simulink model "aocs_plant"  (R2025a)
settings: Solver=ode45  StartTime=0  StopTime=200  RelTol=1e-09  AbsTol=1e-10
undefined symbols (not defined in the file): AOCS, AOCS_Config, AOCS_EnvironmentConfig, AOCS_GNCConfig, AOCS_OrbitConfig, AOCS_SensorConfig, IAU, juliandate, propagateOnboardSgp4
libraries: aerolibtransform2 x8, simulink x8, matrix_library x5
(part 1 of 3)
settings Model: Creator=aocs-simulation  LastModifiedBy=juliankazmierski
settings DebuggingCC: UnconnectedInputMsg=error  UnconnectedOutputMsg=error  UnconnectedLineMsg=error

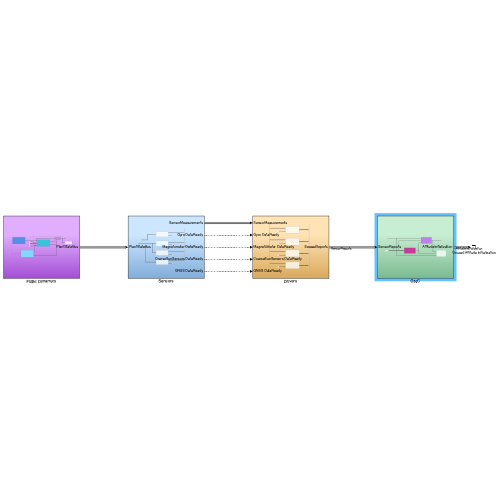
[thumbnail: Simulink's stored preview of the top-level diagram]
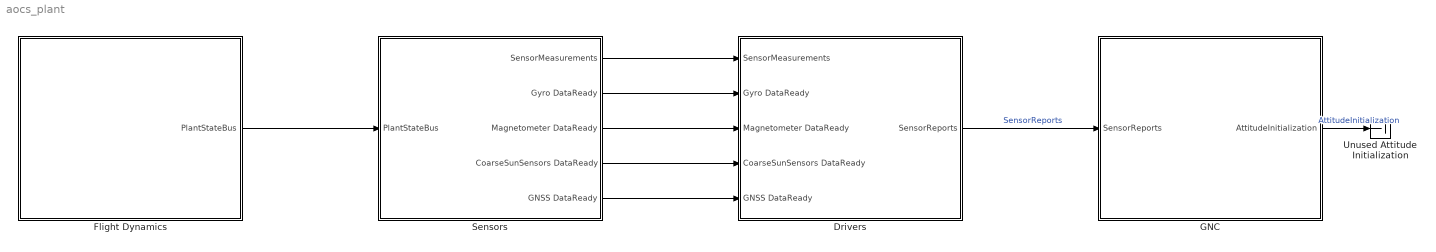
== system aocs_plant ==
  Drivers : Subsystem
  Flight Dynamics : Subsystem
  GNC : Subsystem
  Sensors : Subsystem
  Unused Attitude Initialization : Terminator
  wires:
  Flight Dynamics/1(PlantStateBus) -> Sensors/1(PlantStateBus)
  Sensors/1(SensorMeasurements) -> Drivers/1(SensorMeasurements)
  Sensors/2(Gyro DataReady) -> Drivers/2(Gyro DataReady)
  Sensors/3(Magnetometer DataReady) -> Drivers/3(Magnetometer DataReady)
  Sensors/4(CoarseSunSensors DataReady) -> Drivers/4(CoarseSunSensors DataReady)
  Sensors/5(GNSS DataReady) -> Drivers/5(GNSS DataReady)
  Drivers/1(SensorReports) -> GNC/1(SensorReports)  "SensorReports"
  GNC/1(AttitudeInitialization) -> Unused Attitude Initialization/1  "AttitudeInitialization"

== system aocs_plant/Drivers ==
  SensorMeasurements : Inport  OutDataTypeStr=Bus: SensorMeasurementBus
  Gyro DataReady : Inport  Port=2  OutputFunctionCall=on
  Magnetometer DataReady : Inport  Port=3  OutputFunctionCall=on
  CoarseSunSensors DataReady : Inport  Port=4  OutputFunctionCall=on
  GNSS DataReady : Inport  Port=5  OutputFunctionCall=on
  Coarse Sun Sensors Driver : Subsystem
  GNSS Driver : Subsystem
  Gyro Driver : Subsystem
  Magnetometer Driver : Subsystem
  Select Measurements : BusSelector  OutputSignals=Gyro,Magnetometer,CoarseSunSensors,GNSS
  Sensor Report Bus Assembly : BusCreator  Inputs=4  OutDataTypeStr=Bus: SensorReportBus
  SensorReports : Outport
  wires:
  SensorMeasurements/1 -> Select Measurements/1
  Select Measurements/1 -> Gyro Driver/1(Measurement)  "<Gyro>"
  Gyro DataReady/1 -> Gyro Driver/2(DataReady)
  Select Measurements/2 -> Magnetometer Driver/1(Measurement)  "<Magnetometer>"
  Magnetometer DataReady/1 -> Magnetometer Driver/2(DataReady)
  Select Measurements/3 -> Coarse Sun Sensors Driver/1(Measurement)  "<CoarseSunSensors>"
  CoarseSunSensors DataReady/1 -> Coarse Sun Sensors Driver/2(DataReady)
  Select Measurements/4 -> GNSS Driver/1(Measurement)  "<GNSS>"
  GNSS DataReady/1 -> GNSS Driver/2(DataReady)
  Gyro Driver/1(Report) -> Sensor Report Bus Assembly/1  "Gyro"
  Magnetometer Driver/1(Report) -> Sensor Report Bus Assembly/2  "Magnetometer"
  Coarse Sun Sensors Driver/1(Report) -> Sensor Report Bus Assembly/3  "CoarseSunSensors"
  GNSS Driver/1(Report) -> Sensor Report Bus Assembly/4  "GNSS"
  Sensor Report Bus Assembly/1 -> SensorReports/1

== system aocs_plant/Flight Dynamics ==
  Attitude Dynamics : Subsystem
  Environment Config : Constant  Value=AOCS_EnvironmentConfig  OutDataTypeStr=Bus: EnvironmentConfigBus
  Numerical Checks : Subsystem
  Orbit & Environment : Subsystem
  Orbit Config : Constant  Value=AOCS_OrbitConfig  VectorParams1D=off  OutDataTypeStr=Bus: OrbitConfigBus
  Plant State Bus Creator : BusCreator  Inputs=4  OutDataTypeStr=Bus: PlantStateBus
  Plant Time : Clock
  SpacecraftConfig : Constant  Value=AOCS_Config  OutDataTypeStr=Bus: ConfigBus
  Torque Sum : Subsystem
  PlantStateBus : Outport  OutDataTypeStr=Bus: PlantStateBus
  wires:
  Orbit & Environment/2(EnvironmentBus) -> Torque Sum/2(EnvironmentBus), Plant State Bus Creator/4  "Environment"
  Attitude Dynamics/1(AttitudeState) -> Orbit & Environment/1(AttitudeState), Plant State Bus Creator/3  "AttitudeState"
  Torque Sum/1(Torque_B) -> Attitude Dynamics/1(Torque_B)
  SpacecraftConfig/1 -> Orbit & Environment/4(AocsConfig), Torque Sum/1(Config)
  Environment Config/1 -> Orbit & Environment/3(EnvironmentConfig)
  Orbit Config/1 -> Orbit & Environment/2(OrbitConfig)
  Plant Time/1 -> Plant State Bus Creator/1  "time_s"
  Plant State Bus Creator/1 -> PlantStateBus/1, Numerical Checks/1(PlantState)  "PlantStateBus"
  Orbit & Environment/1(OrbitState) -> Plant State Bus Creator/2  "OrbitState"

== system aocs_plant/GNC ==
  SensorReports : Inport  OutDataTypeStr=Bus: SensorReportBus
  GNC Config : Constant  Value=AOCS_GNCConfig  OutDataTypeStr=Bus: GNCConfigBus
  Onboard Reference Vectors : Subsystem
  Select Initialization Config : BusSelector  OutputSignals=AttitudeInitialization
  State Estimation (MEKF) : Subsystem
  TRIAD Initialization : Subsystem
  AttitudeInitialization : Outport  OutDataTypeStr=Bus: AttitudeInitializationBus
  wires:
  GNC Config/1 -> Select Initialization Config/1
  Select Initialization Config/1 -> Onboard Reference Vectors/1(InitializationConfig), TRIAD Initialization/2(InitializationConfig)  "<AttitudeInitialization>"
  SensorReports/1 -> State Estimation (MEKF)/3(SensorReports), TRIAD Initialization/1(SensorReports)
  Onboard Reference Vectors/1(ReferenceVectors) -> TRIAD Initialization/3(ReferenceVectors), State Estimation (MEKF)/2(ReferenceVectors)  "ReferenceVectors"
  TRIAD Initialization/1(AttitudeInitialization) -> State Estimation (MEKF)/1(AttitudeInitialization), AttitudeInitialization/1  "AttitudeInitialization"

== system aocs_plant/Sensors ==
  PlantStateBus : Inport
  Bus Selector : BusSelector  OutputSignals=AttitudeState,Environment,OrbitState
  Coarse Sun Sensors : Subsystem
  GNSS : Subsystem
  Gyro : Subsystem
  Magnetometer : Subsystem
  Sensor Measurement Bus Assembly : BusCreator  Inputs=4  OutDataTypeStr=Bus: SensorMeasurementBus
  SensorMeasurements : Outport
  Gyro DataReady : Outport  Port=2  OutputFunctionCall=on
  Magnetometer DataReady : Outport  Port=3  OutputFunctionCall=on
  CoarseSunSensors DataReady : Outport  Port=4  OutputFunctionCall=on
  GNSS DataReady : Outport  Port=5  OutputFunctionCall=on
  wires:
  PlantStateBus/1 -> Bus Selector/1
  Bus Selector/1 -> Gyro/1(AttitudeState)  "<AttitudeState>"
  Bus Selector/2 -> Coarse Sun Sensors/1(Environment), Magnetometer/1(Environment)  "<Environment>"
  Gyro/1(Gyro) -> Sensor Measurement Bus Assembly/1  "Gyro"
  Magnetometer/1(Magnetometer) -> Sensor Measurement Bus Assembly/2  "Magnetometer"
  Sensor Measurement Bus Assembly/1 -> SensorMeasurements/1  "SensorMeasurementBus"
  Coarse Sun Sensors/1(CoarseSunSensors) -> Sensor Measurement Bus Assembly/3  "CoarseSunSensors"
  Bus Selector/3 -> GNSS/1(OrbitState)  "<OrbitState>"
  GNSS/1(GNSS) -> Sensor Measurement Bus Assembly/4  "GNSS"
  Gyro/2(DataReady) -> Gyro DataReady/1
  Magnetometer/2(DataReady) -> Magnetometer DataReady/1
  Coarse Sun Sensors/2(DataReady) -> CoarseSunSensors DataReady/1
  GNSS/2(DataReady) -> GNSS DataReady/1

== system aocs_plant/Drivers/Coarse Sun Sensors Driver ==
  Measurement : Inport  OutDataTypeStr=Bus: CoarseSunSensorMeasurementBus
  DataReady : Inport  Port=2  OutputFunctionCall=on
  Receipt Clock : Clock
  Receive Sample : Subsystem
  Report : Outport
  wires:
  Measurement/1 -> Receive Sample/1(Measurement)
  Receipt Clock/1 -> Receive Sample/2(Receipt Time)
  DataReady/1 -> Receive Sample/Trigger
  Receive Sample/1(Report) -> Report/1

== system aocs_plant/Drivers/GNSS Driver ==
  Measurement : Inport  OutDataTypeStr=Bus: GnssMeasurementBus
  DataReady : Inport  Port=2  OutputFunctionCall=on
  Receipt Clock : Clock
  Receive Sample : Subsystem
  Report : Outport
  wires:
  Measurement/1 -> Receive Sample/1(Measurement)
  Receipt Clock/1 -> Receive Sample/2(Receipt Time)
  DataReady/1 -> Receive Sample/Trigger
  Receive Sample/1(Report) -> Report/1

== system aocs_plant/Drivers/Gyro Driver ==
  Measurement : Inport  OutDataTypeStr=Bus: GyroMeasurementBus
  DataReady : Inport  Port=2  OutputFunctionCall=on
  Receipt Clock : Clock
  Receive Sample : Subsystem
  Report : Outport
  wires:
  Measurement/1 -> Receive Sample/1(Measurement)
  Receipt Clock/1 -> Receive Sample/2(Receipt Time)
  DataReady/1 -> Receive Sample/Trigger
  Receive Sample/1(Report) -> Report/1

== system aocs_plant/Drivers/Magnetometer Driver ==
  Measurement : Inport  OutDataTypeStr=Bus: MagnetometerMeasurementBus
  DataReady : Inport  Port=2  OutputFunctionCall=on
  Receipt Clock : Clock
  Receive Sample : Subsystem
  Report : Outport
  wires:
  Measurement/1 -> Receive Sample/1(Measurement)
  Receipt Clock/1 -> Receive Sample/2(Receipt Time)
  DataReady/1 -> Receive Sample/Trigger
  Receive Sample/1(Report) -> Report/1

== system aocs_plant/Flight Dynamics/Attitude Dynamics ==
  Torque_B : Inport
  6DOF (Quaternion) : EOM6DOFBodyQuat  eul_0=AOCS_Config.euler_BI_0_rad  pm_0=AOCS_Config.omega_BI_B_0  mass_0=3.71  inertia=AOCS_Config.I_B
  Bus Creator : BusCreator  Inputs=4
  Terminator : Terminator
  Terminator1 : Terminator
  Terminator2 : Terminator
  Zero_Forces : Constant  Value=[0;0;0]
  AttitudeState : Outport  OutDataTypeStr=Bus: AttitudeStateBus
  wires:
  Torque_B/1 -> 6DOF (Quaternion)/2
  Zero_Forces/1 -> 6DOF (Quaternion)/1
  6DOF (Quaternion)/1 -> Terminator/1
  6DOF (Quaternion)/2 -> Terminator1/1
  6DOF (Quaternion)/6 -> Terminator2/1
  6DOF (Quaternion)/3 -> Bus Creator/1  "euler_rad"
  6DOF (Quaternion)/5 -> Bus Creator/3  "DCM_be"
  6DOF (Quaternion)/7 -> Bus Creator/4  "omega_b"
  Bus Creator/1 -> AttitudeState/1
  6DOF (Quaternion)/4 -> Bus Creator/2  "q_be"

== system aocs_plant/Flight Dynamics/Numerical Checks ==
  PlantState : Inport  OutDataTypeStr=Bus: PlantStateBus
  Finite Plant State : Assertion
  Finite Values : MATLAB Function  TreatAsAtomicUnit=on
  wires:
  PlantState/1 -> Finite Values/1(state)
  Finite Values/1(ok) -> Finite Plant State/1

== system aocs_plant/Flight Dynamics/Orbit & Environment ==
  AttitudeState : Inport
  OrbitConfig : Inport  Port=2
  EnvironmentConfig : Inport  Port=3
  AocsConfig : Inport  Port=4
  Disturbance Torques : Subsystem
  Environment Bus Assembly : Subsystem
  Environment Products : Subsystem
  Orbit Propagator & Time : Subsystem
  OrbitState : Outport  OutDataTypeStr=Bus: OrbitStateBus
  EnvironmentBus : Outport  Port=2  OutDataTypeStr=Bus: EnvironmentBus
  wires:
  AocsConfig/1 -> Disturbance Torques/1(AocsConfig)  "AocsConfig"
  Disturbance Torques/1(Disturbance) -> Environment Bus Assembly/1(Disturbance)  "Disturbance"
  Environment Bus Assembly/1(EnvironmentBus) -> EnvironmentBus/1  "EnvironmentBus"
  Environment Products/2(MagneticField) -> Environment Bus Assembly/2(MagneticField), Disturbance Torques/7(MagneticField)
  AttitudeState/1 -> Disturbance Torques/3(AttitudeState), Environment Products/2(AttitudeState)  "AttitudeState"
  Orbit Propagator & Time/1(OrbitState) -> OrbitState/1, Disturbance Torques/4(OrbitState), Environment Products/3(OrbitState)
  Orbit Propagator & Time/2(EnvironmentContext) -> Disturbance Torques/5(EnvironmentContext), Environment Products/4(EnvironmentContext)
  EnvironmentConfig/1 -> Environment Products/1(EnvironmentConfig), Disturbance Torques/2(EnvironmentConfig)  "EnvironmentConfig"
  Environment Products/1(SRP) -> Disturbance Torques/6(SRP)
  Environment Products/4(Illumination) -> Environment Bus Assembly/4(Illumination)
  Environment Products/3(Sun) -> Environment Bus Assembly/3(Sun)
  OrbitConfig/1 -> Orbit Propagator & Time/1(OrbitConfig)  "OrbitConfig"
  Environment Products/5(Atmosphere) -> Disturbance Torques/8(Atmosphere), Environment Bus Assembly/5(Atmosphere)
  Disturbance Torques/2(OrbitAcceleration) -> Orbit Propagator & Time/2(OrbitAcceleration)

== system aocs_plant/Flight Dynamics/Torque Sum ==
  Config : Inport
  EnvironmentBus : Inport  Port=2
  Add : Sum
  Bus Selector : BusSelector  OutputSignals=M_dist_B_Nm
  Bus Selector1 : BusSelector  OutputSignals=M_ext_B
  Torque_B : Outport
  wires:
  EnvironmentBus/1 -> Bus Selector/1
  Bus Selector/1 -> Add/1  "<M_dist_B_Nm>"
  Add/1 -> Torque_B/1
  Config/1 -> Bus Selector1/1
  Bus Selector1/1 -> Add/2  "<M_ext_B>"

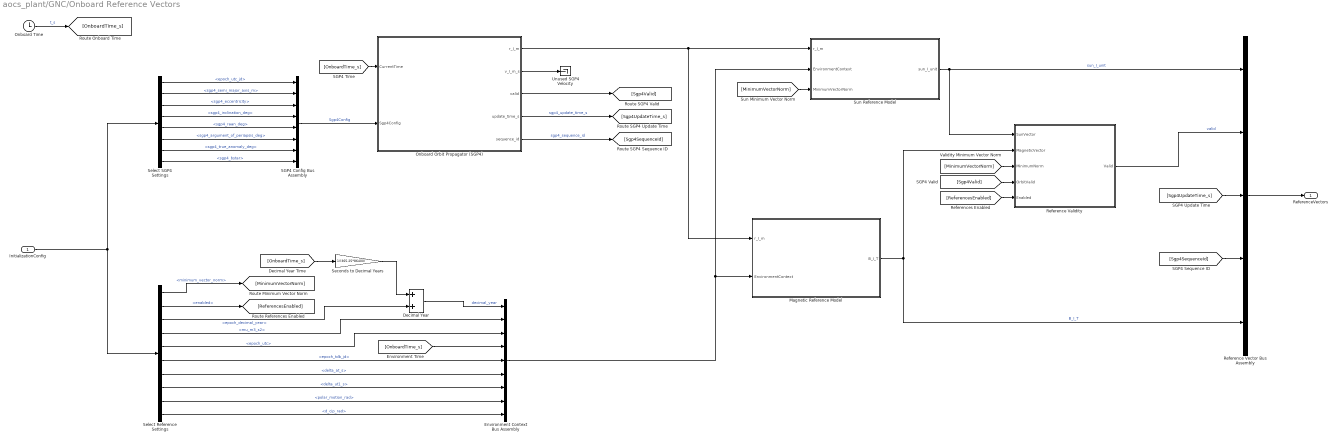
== system aocs_plant/GNC/Onboard Reference Vectors ==
  InitializationConfig : Inport  OutDataTypeStr=Bus: AttitudeInitializationConfigBus
  Decimal Year : Sum
  Environment Context Bus Assembly : BusCreator  Inputs=9  OutDataTypeStr=Bus: EnvironmentContextBus
  Magnetic Reference Model : Subsystem
  Onboard Orbit Propagator (SGP4) : Subsystem
  Onboard Time : Clock
  Reference Validity : Subsystem
  Reference Vector Bus Assembly : BusCreator  Inputs=5  OutDataTypeStr=Bus: ReferenceVectorBus
  SGP4 Config Bus Assembly : BusCreator  Inputs=8  OutDataTypeStr=Bus: Sgp4ConfigBus  NonVirtualBus=on
  Seconds to Decimal Years : Gain  Gain=1/(365.25*86400)
  Select Reference Settings : BusSelector  OutputSignals=minimum_vector_norm,enabled,epoch_decimal_year,mu_m3_s2,epoch_utc,epoch_tdb_jd,delta_at_s,delta_ut1_s,polar_motion_rad,d_cip_rad
  Select SGP4 Settings : BusSelector  OutputSignals=epoch_utc_jd,sgp4_semi_major_axis_m,sgp4_eccentricity,sgp4_inclination_deg,sgp4_raan_deg,sgp4_argument_of_periapsis_deg,sgp4_true_anomaly_deg,sgp4_bstar
  Sun Reference Model : Subsystem
  Unused SGP4 Velocity : Terminator
  ReferenceVectors : Outport  OutDataTypeStr=Bus: ReferenceVectorBus
  wires:
  InitializationConfig/1 -> Select Reference Settings/1, Select SGP4 Settings/1
  Onboard Time/1 -> [OnboardTime_s]  "t_s"
  Select SGP4 Settings/1 -> SGP4 Config Bus Assembly/1  "<epoch_utc_jd>"
  Select SGP4 Settings/2 -> SGP4 Config Bus Assembly/2  "<sgp4_semi_major_axis_m>"
  Select SGP4 Settings/3 -> SGP4 Config Bus Assembly/3  "<sgp4_eccentricity>"
  Select SGP4 Settings/4 -> SGP4 Config Bus Assembly/4  "<sgp4_inclination_deg>"
  Select SGP4 Settings/5 -> SGP4 Config Bus Assembly/5  "<sgp4_raan_deg>"
  Select SGP4 Settings/6 -> SGP4 Config Bus Assembly/6  "<sgp4_argument_of_periapsis_deg>"
  Select SGP4 Settings/7 -> SGP4 Config Bus Assembly/7  "<sgp4_true_anomaly_deg>"
  Select SGP4 Settings/8 -> SGP4 Config Bus Assembly/8  "<sgp4_bstar>"
  [OnboardTime_s] -> Onboard Orbit Propagator (SGP4)/1(CurrentTime)
  SGP4 Config Bus Assembly/1 -> Onboard Orbit Propagator (SGP4)/2(Sgp4Config)  "Sgp4Config"
  Select Reference Settings/1 -> [MinimumVectorNorm]  "<minimum_vector_norm>"
  Select Reference Settings/2 -> [ReferencesEnabled]  "<enabled>"
  Select Reference Settings/3 -> Decimal Year/2  "<epoch_decimal_year>"
  Select Reference Settings/4 -> Environment Context Bus Assembly/2  "<mu_m3_s2>"
  Select Reference Settings/5 -> Environment Context Bus Assembly/3  "<epoch_utc>"
  Select Reference Settings/6 -> Environment Context Bus Assembly/5  "<epoch_tdb_jd>"
  Select Reference Settings/7 -> Environment Context Bus Assembly/6  "<delta_at_s>"
  Select Reference Settings/8 -> Environment Context Bus Assembly/7  "<delta_ut1_s>"
  Select Reference Settings/9 -> Environment Context Bus Assembly/8  "<polar_motion_rad>"
  Select Reference Settings/10 -> Environment Context Bus Assembly/9  "<d_cip_rad>"
  [OnboardTime_s] -> Seconds to Decimal Years/1
  Seconds to Decimal Years/1 -> Decimal Year/1
  Decimal Year/1 -> Environment Context Bus Assembly/1  "decimal_year"
  [OnboardTime_s] -> Environment Context Bus Assembly/4
  Onboard Orbit Propagator (SGP4)/1(r_I_m) -> Sun Reference Model/1(r_I_m), Magnetic Reference Model/1(r_I_m)
  Onboard Orbit Propagator (SGP4)/2(v_I_m_s) -> Unused SGP4 Velocity/1
  Onboard Orbit Propagator (SGP4)/3(valid) -> [Sgp4Valid]
  Onboard Orbit Propagator (SGP4)/4(update_time_s) -> [Sgp4UpdateTime_s]  "sgp4_update_time_s"
  Onboard Orbit Propagator (SGP4)/5(sequence_id) -> [Sgp4SequenceId]  "sgp4_sequence_id"
  Environment Context Bus Assembly/1 -> Magnetic Reference Model/2(EnvironmentContext), Sun Reference Model/2(EnvironmentContext)
  [MinimumVectorNorm] -> Sun Reference Model/3(MinimumVectorNorm)
  Sun Reference Model/1(sun_I_unit) -> Reference Validity/1(SunVector), Reference Vector Bus Assembly/1  "sun_I_unit"
  Magnetic Reference Model/1(B_I_T) -> Reference Vector Bus Assembly/5, Reference Validity/2(MagneticVector)  "B_I_T"
  [MinimumVectorNorm] -> Reference Validity/3(MinimumNorm)
  [Sgp4Valid] -> Reference Validity/4(OrbitValid)
  [ReferencesEnabled] -> Reference Validity/5(Enabled)
  Reference Validity/1(Valid) -> Reference Vector Bus Assembly/2  "valid"
  [Sgp4UpdateTime_s] -> Reference Vector Bus Assembly/3
  [Sgp4SequenceId] -> Reference Vector Bus Assembly/4
  Reference Vector Bus Assembly/1 -> ReferenceVectors/1

== system aocs_plant/GNC/State Estimation (MEKF) ==
  note: Reserved for the six-state multiplicative EKF: attitude error plus gyro bias.
  AttitudeInitialization : Inport  OutDataTypeStr=Bus: AttitudeInitializationBus
  ReferenceVectors : Inport  Port=2  OutDataTypeStr=Bus: ReferenceVectorBus
  SensorReports : Inport  Port=3  OutDataTypeStr=Bus: SensorReportBus
  Unused AttitudeInitialization : Terminator
  Unused ReferenceVectors : Terminator
  Unused SensorReports : Terminator
  wires:
  SensorReports/1 -> Unused SensorReports/1
  ReferenceVectors/1 -> Unused ReferenceVectors/1
  AttitudeInitialization/1 -> Unused AttitudeInitialization/1

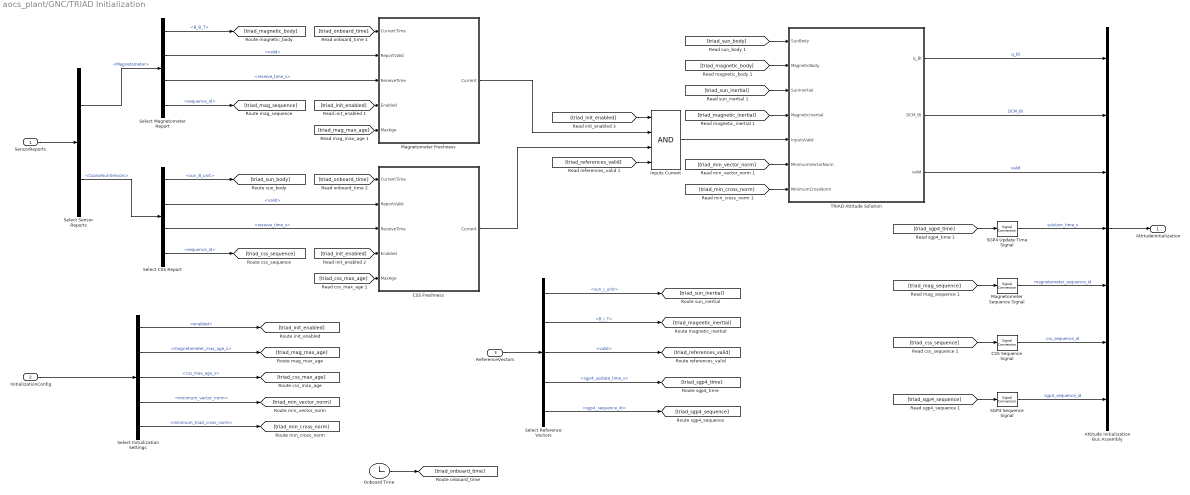
== system aocs_plant/GNC/TRIAD Initialization ==
  SensorReports : Inport  OutDataTypeStr=Bus: SensorReportBus
  InitializationConfig : Inport  Port=2  OutDataTypeStr=Bus: AttitudeInitializationConfigBus
  ReferenceVectors : Inport  Port=3  OutDataTypeStr=Bus: ReferenceVectorBus
  Attitude Initialization Bus Assembly : BusCreator  Inputs=7  OutDataTypeStr=Bus: AttitudeInitializationBus
  CSS Freshness : Subsystem
  CSS Sequence Signal : SignalConversion  OverrideOpt=off
  Inputs Current : Logic  Inputs=4  AllPortsSameDT=off  OutDataTypeStr=boolean
  Magnetometer Freshness : Subsystem
  Magnetometer Sequence Signal : SignalConversion  OverrideOpt=off
  Onboard Time : Clock
  SGP4 Sequence Signal : SignalConversion  OverrideOpt=off
  SGP4 Update Time Signal : SignalConversion  OverrideOpt=off
  Select CSS Report : BusSelector  OutputSignals=sun_B_unit,valid,receive_time_s,sequence_id
  Select Initialization Settings : BusSelector  OutputSignals=enabled,magnetometer_max_age_s,css_max_age_s,minimum_vector_norm,minimum_triad_cross_norm
  Select Magnetometer Report : BusSelector  OutputSignals=B_B_T,valid,receive_time_s,sequence_id
  Select Reference Vectors : BusSelector  OutputSignals=sun_I_unit,B_I_T,valid,sgp4_update_time_s,sgp4_sequence_id
  Select Sensor Reports : BusSelector  OutputSignals=Magnetometer,CoarseSunSensors
  TRIAD Attitude Solution : Subsystem
  AttitudeInitialization : Outport  OutDataTypeStr=Bus: AttitudeInitializationBus
  wires:
  SensorReports/1 -> Select Sensor Reports/1
  Select Sensor Reports/1 -> Select Magnetometer Report/1  "<Magnetometer>"
  Select Sensor Reports/2 -> Select CSS Report/1  "<CoarseSunSensors>"
  ReferenceVectors/1 -> Select Reference Vectors/1
  InitializationConfig/1 -> Select Initialization Settings/1
  Select Magnetometer Report/2 -> Magnetometer Freshness/2(ReportValid)  "<valid>"
  Select Magnetometer Report/3 -> Magnetometer Freshness/3(ReceiveTime)  "<receive_time_s>"
  Select CSS Report/2 -> CSS Freshness/2(ReportValid)  "<valid>"
  Select CSS Report/3 -> CSS Freshness/3(ReceiveTime)  "<receive_time_s>"
  Magnetometer Freshness/1(Current) -> Inputs Current/2
  CSS Freshness/1(Current) -> Inputs Current/3
  Inputs Current/1 -> TRIAD Attitude Solution/5(InputsValid)
  TRIAD Attitude Solution/1(q_BI) -> Attitude Initialization Bus Assembly/1  "q_BI"
  TRIAD Attitude Solution/2(DCM_BI) -> Attitude Initialization Bus Assembly/2  "DCM_BI"
  TRIAD Attitude Solution/3(valid) -> Attitude Initialization Bus Assembly/3  "valid"
  SGP4 Update Time Signal/1 -> Attitude Initialization Bus Assembly/4  "solution_time_s"
  Magnetometer Sequence Signal/1 -> Attitude Initialization Bus Assembly/5  "magnetometer_sequence_id"
  CSS Sequence Signal/1 -> Attitude Initialization Bus Assembly/6  "css_sequence_id"
  SGP4 Sequence Signal/1 -> Attitude Initialization Bus Assembly/7  "sgp4_sequence_id"
  Attitude Initialization Bus Assembly/1 -> AttitudeInitialization/1
  Select Magnetometer Report/1 -> [triad_magnetic_body]  "<B_B_T>"
  [triad_magnetic_body] -> TRIAD Attitude Solution/2(MagneticBody)
  Select Magnetometer Report/4 -> [triad_mag_sequence]  "<sequence_id>"
  [triad_mag_sequence] -> Magnetometer Sequence Signal/1
  Select CSS Report/1 -> [triad_sun_body]  "<sun_B_unit>"
  [triad_sun_body] -> TRIAD Attitude Solution/1(SunBody)
  Select CSS Report/4 -> [triad_css_sequence]  "<sequence_id>"
  [triad_css_sequence] -> CSS Sequence Signal/1
  Select Initialization Settings/1 -> [triad_init_enabled]  "<enabled>"
  [triad_init_enabled] -> Magnetometer Freshness/4(Enabled)
  [triad_init_enabled] -> CSS Freshness/4(Enabled)
  [triad_init_enabled] -> Inputs Current/1
  Select Initialization Settings/2 -> [triad_mag_max_age]  "<magnetometer_max_age_s>"
  [triad_mag_max_age] -> Magnetometer Freshness/5(MaxAge)
  Select Initialization Settings/3 -> [triad_css_max_age]  "<css_max_age_s>"
  [triad_css_max_age] -> CSS Freshness/5(MaxAge)
  Select Initialization Settings/4 -> [triad_min_vector_norm]  "<minimum_vector_norm>"
  [triad_min_vector_norm] -> TRIAD Attitude Solution/6(MinimumVectorNorm)
  Select Initialization Settings/5 -> [triad_min_cross_norm]  "<minimum_triad_cross_norm>"
  [triad_min_cross_norm] -> TRIAD Attitude Solution/7(MinimumCrossNorm)
  Select Reference Vectors/1 -> [triad_sun_inertial]  "<sun_I_unit>"
  [triad_sun_inertial] -> TRIAD Attitude Solution/3(SunInertial)
  Select Reference Vectors/2 -> [triad_magnetic_inertial]  "<B_I_T>"
  [triad_magnetic_inertial] -> TRIAD Attitude Solution/4(MagneticInertial)
  Select Reference Vectors/3 -> [triad_references_valid]  "<valid>"
  [triad_references_valid] -> Inputs Current/4
  Select Reference Vectors/4 -> [triad_sgp4_time]  "<sgp4_update_time_s>"
  [triad_sgp4_time] -> SGP4 Update Time Signal/1
  Select Reference Vectors/5 -> [triad_sgp4_sequence]  "<sgp4_sequence_id>"
  [triad_sgp4_sequence] -> SGP4 Sequence Signal/1
  Onboard Time/1 -> [triad_onboard_time]
  [triad_onboard_time] -> Magnetometer Freshness/1(CurrentTime)
  [triad_onboard_time] -> CSS Freshness/1(CurrentTime)

== system aocs_plant/Sensors/Coarse Sun Sensors ==
  Environment : Inport
  Bus Selector : BusSelector  OutputSignals=sun_B_unit,solar_flux_shadowed_W_m2,sun_visibility
  CSS Measurement Bus Assembly : BusCreator  Inputs=4  OutDataTypeStr=Bus: CoarseSunSensorMeasurementBus
  Coarse Sun Sensor Model : MATLAB Function  TreatAsAtomicUnit=on
  CssConfig : Constant  Value=AOCS_SensorConfig.CoarseSunSensors  OutDataTypeStr=Bus: CoarseSunSensorConfigBus
  DataReady Generator : FunctionCallGenerator  SampleTime=AOCS_SensorConfig.CoarseSunSensors.sample_time_s
  Measurement Sample Hold : ZeroOrderHold  SampleTime=AOCS_SensorConfig.CoarseSunSensors.sample_time_s
  W : RandomNumber  Mean=zeros(6,1)  Variance=ones(6,1)  Seed=AOCS_SensorConfig.CoarseSunSensors.noise_seed  SampleTime=AOCS_SensorConfig.CoarseSunSensors.sample_time_s
  CoarseSunSensors : Outport
  DataReady : Outport  Port=2  OutputFunctionCall=on
  wires:
  Environment/1 -> Bus Selector/1
  Bus Selector/1 -> Coarse Sun Sensor Model/1(sun_B_unit)  "<sun_B_unit>"
  Bus Selector/2 -> Coarse Sun Sensor Model/2(solar_flux_shadowed_W_m2)  "<solar_flux_shadowed_W_m2>"
  Bus Selector/3 -> Coarse Sun Sensor Model/3(sun_visibility)  "<sun_visibility>"
  CssConfig/1 -> Coarse Sun Sensor Model/4(css)  "css"
  W/1 -> Coarse Sun Sensor Model/5(noise_unit)  "noise_unit"
  Coarse Sun Sensor Model/1(sun_B_unit_meas) -> CSS Measurement Bus Assembly/1  "sun_B_unit"
  Coarse Sun Sensor Model/2(irradiance_W_m2) -> CSS Measurement Bus Assembly/2  "irradiance_W_m2"
  Coarse Sun Sensor Model/3(panel_signals_W_m2) -> CSS Measurement Bus Assembly/3  "panel_signals_W_m2"
  Coarse Sun Sensor Model/4(valid) -> CSS Measurement Bus Assembly/4  "valid"
  CSS Measurement Bus Assembly/1 -> Measurement Sample Hold/1  "CoarseSunSensors"
  Measurement Sample Hold/1 -> CoarseSunSensors/1
  DataReady Generator/1 -> DataReady/1

== system aocs_plant/Sensors/GNSS ==
  OrbitState : Inport
  DataReady Generator : FunctionCallGenerator  SampleTime=AOCS_SensorConfig.GNSS.sample_time_s
  Fix Availability : Subsystem
  GNSS Measurement Bus Assembly : BusCreator  Inputs=3  OutDataTypeStr=Bus: GnssMeasurementBus
  GnssConfig : Constant  Value=AOCS_SensorConfig.GNSS  OutDataTypeStr=Bus: GnssConfigBus
  Measurement Sample Hold : ZeroOrderHold  SampleTime=AOCS_SensorConfig.GNSS.sample_time_s
  Output Selection : Subsystem
  PVT Error Model : Subsystem
  Position Quantizer : Quantizer  QuantizationInterval=AOCS_SensorConfig.GNSS.position_resolution_m
  Position Sample Hold : ZeroOrderHold  SampleTime=AOCS_SensorConfig.GNSS.sample_time_s
  Select Orbit State : BusSelector  OutputSignals=r_I_m,v_I_m_s
  Velocity Quantizer : Quantizer  QuantizationInterval=AOCS_SensorConfig.GNSS.velocity_resolution_m_s
  Velocity Sample Hold : ZeroOrderHold  SampleTime=AOCS_SensorConfig.GNSS.sample_time_s
  GNSS : Outport
  DataReady : Outport  Port=2  OutputFunctionCall=on
  wires:
  OrbitState/1 -> Select Orbit State/1  "OrbitState"
  Select Orbit State/1 -> Position Sample Hold/1  "<r_I_m>"
  Select Orbit State/2 -> Velocity Sample Hold/1  "<v_I_m_s>"
  Position Sample Hold/1 -> PVT Error Model/1(rTruth_I_m)
  Velocity Sample Hold/1 -> PVT Error Model/2(vTruth_I_m_s)
  PVT Error Model/1(rMeasured_I_m) -> Position Quantizer/1
  PVT Error Model/2(vMeasured_I_m_s) -> Velocity Quantizer/1
  Position Quantizer/1 -> Output Selection/1(rNominal_I_m)  "r_I_m_nominal"
  Velocity Quantizer/1 -> Output Selection/2(vNominal_I_m_s)  "v_I_m_s_nominal"
  GnssConfig/1 -> Fix Availability/1(GnssConfig), Output Selection/3(GnssConfig)  "GNSSConfig"
  Fix Availability/1(fix_available) -> Output Selection/4(fix_available)  "fix_available"
  Output Selection/1(r_I_m) -> GNSS Measurement Bus Assembly/1  "r_I_m"
  Output Selection/2(v_I_m_s) -> GNSS Measurement Bus Assembly/2  "v_I_m_s"
  Output Selection/3(valid) -> GNSS Measurement Bus Assembly/3  "valid"
  GNSS Measurement Bus Assembly/1 -> Measurement Sample Hold/1  "GNSS"
  Measurement Sample Hold/1 -> GNSS/1
  DataReady Generator/1 -> DataReady/1

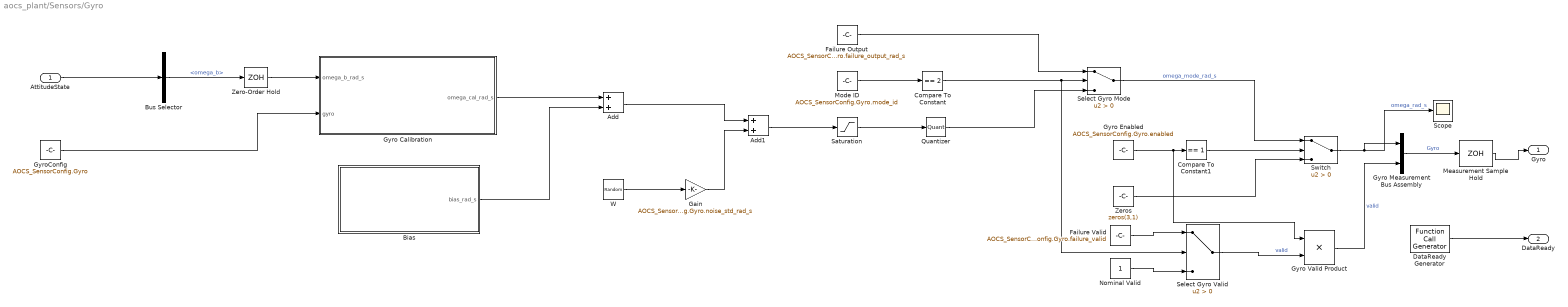
== system aocs_plant/Sensors/Gyro ==
  AttitudeState : Inport
  Add : Sum
  Add1 : Sum
  Bias : Subsystem
  Bus Selector : BusSelector  OutputSignals=omega_b
  Compare To Constant : simulink/Logic and Bit Operations/Compare To Constant  relop===  const=2  OutDataTypeStr=boolean
  Compare To Constant1 : simulink/Logic and Bit Operations/Compare To Constant  relop===  const=1  OutDataTypeStr=boolean
  DataReady Generator : FunctionCallGenerator  SampleTime=AOCS_SensorConfig.Gyro.gyro_sample_time_s
  Failure Output : Constant  Value=AOCS_SensorConfig.Gyro.failure_output_rad_s
  Failure Valid : Constant  Value=AOCS_SensorConfig.Gyro.failure_valid
  Gain : Gain  Gain=AOCS_SensorConfig.Gyro.noise_std_rad_s
  Gyro Calibration : MATLAB Function  TreatAsAtomicUnit=on
  Gyro Enabled : Constant  Value=AOCS_SensorConfig.Gyro.enabled
  Gyro Measurement Bus Assembly : BusCreator  Inputs=2  OutDataTypeStr=Bus: GyroMeasurementBus
  Gyro Valid Product : Product  Inputs=**
  GyroConfig : Constant  Value=AOCS_SensorConfig.Gyro  OutDataTypeStr=Bus: GyroConfigBus
  Measurement Sample Hold : ZeroOrderHold  SampleTime=AOCS_SensorConfig.Gyro.gyro_sample_time_s
  Mode ID : Constant  Value=AOCS_SensorConfig.Gyro.mode_id
  Nominal Valid : Constant
  Quantizer : Quantizer  QuantizationInterval=AOCS_SensorConfig.Gyro.resolution_rad_s
  Saturation : Saturate  UpperLimit=AOCS_SensorConfig.Gyro.range_rad_s  LowerLimit=-AOCS_SensorConfig.Gyro.range_rad_s
  Scope : Scope
      settings: ActiveDisplayYMinimum=1.4855983316703409  ActiveDisplayYMaximum=1.511725104472023
  Select Gyro Mode : Switch  Criteria=u2 > Threshold  SaturateOnIntegerOverflow=off  InputSameDT=off
  Select Gyro Valid : Switch  Criteria=u2 > Threshold  SaturateOnIntegerOverflow=off  InputSameDT=off
  Switch : Switch  Criteria=u2 > Threshold  SaturateOnIntegerOverflow=off  InputSameDT=off
  W : RandomNumber  Seed=AOCS_SensorConfig.Gyro.noise_seed  SampleTime=AOCS_SensorConfig.Gyro.gyro_sample_time_s
  Zero-Order Hold : ZeroOrderHold  SampleTime=AOCS_SensorConfig.Gyro.gyro_sample_time_s
  Zeros : Constant  Value=zeros(3,1)
  Gyro : Outport
  DataReady : Outport  Port=2  OutputFunctionCall=on
  wires:
  AttitudeState/1 -> Bus Selector/1
  Bus Selector/1 -> Zero-Order Hold/1  "<omega_b>"
  Zero-Order Hold/1 -> Gyro Calibration/1(omega_b_rad_s)
  GyroConfig/1 -> Gyro Calibration/2(gyro)
  Gyro Calibration/1(omega_cal_rad_s) -> Add/1
  Bias/1(bias_rad_s) -> Add/2
  W/1 -> Gain/1
  Gain/1 -> Add1/2
  Add/1 -> Add1/1
  Add1/1 -> Saturation/1
  Saturation/1 -> Quantizer/1
  Mode ID/1 -> Compare To Constant/1
  Compare To Constant/1 -> Select Gyro Mode/2, Select Gyro Valid/2
  Failure Output/1 -> Select Gyro Mode/1
  Quantizer/1 -> Select Gyro Mode/3
  Select Gyro Mode/1 -> Switch/1  "omega_mode_rad_s"
  Gyro Enabled/1 -> Compare To Constant1/1, Gyro Valid Product/1
  Compare To Constant1/1 -> Switch/2
  Zeros/1 -> Switch/3
  Switch/1 -> Scope/1, Gyro Measurement Bus Assembly/1  "omega_rad_s"
  Failure Valid/1 -> Select Gyro Valid/1
  Nominal Valid/1 -> Select Gyro Valid/3
  Select Gyro Valid/1 -> Gyro Valid Product/2  "valid"
  Gyro Valid Product/1 -> Gyro Measurement Bus Assembly/2  "valid"
  Gyro Measurement Bus Assembly/1 -> Measurement Sample Hold/1  "Gyro"
  Measurement Sample Hold/1 -> Gyro/1
  DataReady Generator/1 -> DataReady/1

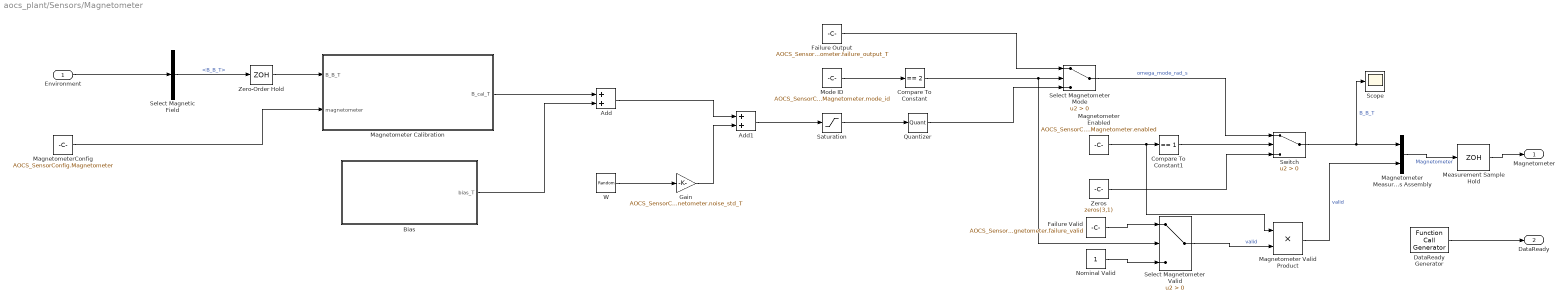
== system aocs_plant/Sensors/Magnetometer ==
  Environment : Inport
  Add : Sum
  Add1 : Sum
  Bias : Subsystem
  Compare To Constant : simulink/Logic and Bit Operations/Compare To Constant  relop===  const=2  OutDataTypeStr=boolean
  Compare To Constant1 : simulink/Logic and Bit Operations/Compare To Constant  relop===  const=1  OutDataTypeStr=boolean
  DataReady Generator : FunctionCallGenerator  SampleTime=AOCS_SensorConfig.Magnetometer.sample_time_s
  Failure Output : Constant  Value=AOCS_SensorConfig.Magnetometer.failure_output_T
  Failure Valid : Constant  Value=AOCS_SensorConfig.Magnetometer.failure_valid
  Gain : Gain  Gain=AOCS_SensorConfig.Magnetometer.noise_std_T
  Magnetometer Calibration : MATLAB Function  TreatAsAtomicUnit=on
  Magnetometer Enabled : Constant  Value=AOCS_SensorConfig.Magnetometer.enabled
  Magnetometer Measurement Bus Assembly : BusCreator  Inputs=2  OutDataTypeStr=Bus: MagnetometerMeasurementBus
  Magnetometer Valid Product : Product  Inputs=**
  MagnetometerConfig : Constant  Value=AOCS_SensorConfig.Magnetometer  OutDataTypeStr=Bus: MagnetometerConfigBus
  Measurement Sample Hold : ZeroOrderHold  SampleTime=AOCS_SensorConfig.Magnetometer.sample_time_s
  Mode ID : Constant  Value=AOCS_SensorConfig.Magnetometer.mode_id
  Nominal Valid : Constant
  Quantizer : Quantizer  QuantizationInterval=AOCS_SensorConfig.Magnetometer.resolution_T
  Saturation : Saturate  UpperLimit=AOCS_SensorConfig.Magnetometer.range_T  LowerLimit=-AOCS_SensorConfig.Magnetometer.range_T
  Scope : Scope
      settings: ActiveDisplayYMinimum=0.99973136391270112  ActiveDisplayYMaximum=1.0056523225715319
  Select Magnetic Field : BusSelector  OutputSignals=B_B_T
  Select Magnetometer Mode : Switch  Criteria=u2 > Threshold  SaturateOnIntegerOverflow=off  InputSameDT=off
  Select Magnetometer Valid : Switch  Criteria=u2 > Threshold  SaturateOnIntegerOverflow=off  InputSameDT=off
  Switch : Switch  Criteria=u2 > Threshold  SaturateOnIntegerOverflow=off  InputSameDT=off
  W : RandomNumber  Seed=AOCS_SensorConfig.Magnetometer.noise_seed  SampleTime=AOCS_SensorConfig.Magnetometer.sample_time_s
  Zero-Order Hold : ZeroOrderHold  SampleTime=AOCS_SensorConfig.Magnetometer.sample_time_s
  Zeros : Constant  Value=zeros(3,1)
  Magnetometer : Outport
  DataReady : Outport  Port=2  OutputFunctionCall=on
  wires:
  Magnetometer Valid Product/1 -> Magnetometer Measurement Bus Assembly/2  "valid"
  Select Magnetometer Valid/1 -> Magnetometer Valid Product/2  "valid"
  Nominal Valid/1 -> Select Magnetometer Valid/3
  Failure Valid/1 -> Select Magnetometer Valid/1
  Zeros/1 -> Switch/3
  Compare To Constant1/1 -> Switch/2
  Magnetometer Enabled/1 -> Magnetometer Valid Product/1, Compare To Constant1/1
  Select Magnetometer Mode/1 -> Switch/1  "omega_mode_rad_s"
  Quantizer/1 -> Select Magnetometer Mode/3
  Failure Output/1 -> Select Magnetometer Mode/1
  Compare To Constant/1 -> Select Magnetometer Valid/2, Select Magnetometer Mode/2
  Mode ID/1 -> Compare To Constant/1
  Saturation/1 -> Quantizer/1
  Add1/1 -> Saturation/1
  Add/1 -> Add1/1
  Gain/1 -> Add1/2
  W/1 -> Gain/1
  Bias/1(bias_T) -> Add/2
  Magnetometer Calibration/1(B_cal_T) -> Add/1
  MagnetometerConfig/1 -> Magnetometer Calibration/2(magnetometer)
  Zero-Order Hold/1 -> Magnetometer Calibration/1(B_B_T)
  Select Magnetic Field/1 -> Zero-Order Hold/1  "<B_B_T>"
  Environment/1 -> Select Magnetic Field/1
  Switch/1 -> Scope/1, Magnetometer Measurement Bus Assembly/1  "B_B_T"
  Magnetometer Measurement Bus Assembly/1 -> Measurement Sample Hold/1  "Magnetometer"
  Measurement Sample Hold/1 -> Magnetometer/1
  DataReady Generator/1 -> DataReady/1

== system aocs_plant/Drivers/Coarse Sun Sensors Driver/Receive Sample ==
  Measurement : Inport  OutDataTypeStr=Bus: CoarseSunSensorMeasurementBus
  Receipt Time : Inport  Port=2
  DataReady : TriggerPort  TriggerType=function-call  VariantControl=(inherit)  PortDimensions=1
  Last Sequence : UnitDelay  InitialCondition=uint32(0)  SampleTime=-1  HasFrameUpgradeWarning=on
  Next Sequence : Sum  OutDataTypeStr=uint32
  One : Constant  Value=uint32(1)  OutDataTypeStr=uint32
  Payload : BusSelector  OutputSignals=sun_B_unit,irradiance_W_m2,panel_signals_W_m2,valid
  Report Assembly : BusCreator  Inputs=6  OutDataTypeStr=Bus: CoarseSunSensorReportBus  NonVirtualBus=on
  Report : Outport  InitialOutput=0
  wires:
  Measurement/1 -> Payload/1
  Payload/1 -> Report Assembly/1  "<sun_B_unit>"
  Payload/2 -> Report Assembly/2  "<irradiance_W_m2>"
  Payload/3 -> Report Assembly/3  "<panel_signals_W_m2>"
  Payload/4 -> Report Assembly/4  "<valid>"
  Receipt Time/1 -> Report Assembly/5  "receive_time_s"
  Last Sequence/1 -> Next Sequence/1
  One/1 -> Next Sequence/2
  Next Sequence/1 -> Last Sequence/1, Report Assembly/6  "sequence_id"
  Report Assembly/1 -> Report/1

== system aocs_plant/Drivers/GNSS Driver/Receive Sample ==
  Measurement : Inport  OutDataTypeStr=Bus: GnssMeasurementBus
  Receipt Time : Inport  Port=2
  DataReady : TriggerPort  TriggerType=function-call  VariantControl=(inherit)  PortDimensions=1
  Last Sequence : UnitDelay  InitialCondition=uint32(0)  SampleTime=-1  HasFrameUpgradeWarning=on
  Next Sequence : Sum  OutDataTypeStr=uint32
  One : Constant  Value=uint32(1)  OutDataTypeStr=uint32
  Payload : BusSelector  OutputSignals=r_I_m,v_I_m_s,valid
  Report Assembly : BusCreator  Inputs=5  OutDataTypeStr=Bus: GnssReportBus  NonVirtualBus=on
  Report : Outport  InitialOutput=0
  wires:
  Measurement/1 -> Payload/1
  Payload/1 -> Report Assembly/1  "<r_I_m>"
  Payload/2 -> Report Assembly/2  "<v_I_m_s>"
  Payload/3 -> Report Assembly/3  "<valid>"
  Receipt Time/1 -> Report Assembly/4  "receive_time_s"
  Last Sequence/1 -> Next Sequence/1
  One/1 -> Next Sequence/2
  Next Sequence/1 -> Last Sequence/1, Report Assembly/5  "sequence_id"
  Report Assembly/1 -> Report/1

== system aocs_plant/Drivers/Gyro Driver/Receive Sample ==
  Measurement : Inport  OutDataTypeStr=Bus: GyroMeasurementBus
  Receipt Time : Inport  Port=2
  DataReady : TriggerPort  TriggerType=function-call  VariantControl=(inherit)  PortDimensions=1
  Last Sequence : UnitDelay  InitialCondition=uint32(0)  SampleTime=-1  HasFrameUpgradeWarning=on
  Next Sequence : Sum  OutDataTypeStr=uint32
  One : Constant  Value=uint32(1)  OutDataTypeStr=uint32
  Payload : BusSelector  OutputSignals=omega_rad_s,valid
  Report Assembly : BusCreator  Inputs=4  OutDataTypeStr=Bus: GyroReportBus  NonVirtualBus=on
  Report : Outport  InitialOutput=0
  wires:
  Measurement/1 -> Payload/1
  Payload/1 -> Report Assembly/1  "<omega_rad_s>"
  Payload/2 -> Report Assembly/2  "<valid>"
  Receipt Time/1 -> Report Assembly/3  "receive_time_s"
  Last Sequence/1 -> Next Sequence/1
  One/1 -> Next Sequence/2
  Next Sequence/1 -> Last Sequence/1, Report Assembly/4  "sequence_id"
  Report Assembly/1 -> Report/1

== system aocs_plant/Drivers/Magnetometer Driver/Receive Sample ==
  Measurement : Inport  OutDataTypeStr=Bus: MagnetometerMeasurementBus
  Receipt Time : Inport  Port=2
  DataReady : TriggerPort  TriggerType=function-call  VariantControl=(inherit)  PortDimensions=1
  Last Sequence : UnitDelay  InitialCondition=uint32(0)  SampleTime=-1  HasFrameUpgradeWarning=on
  Next Sequence : Sum  OutDataTypeStr=uint32
  One : Constant  Value=uint32(1)  OutDataTypeStr=uint32
  Payload : BusSelector  OutputSignals=B_B_T,valid
  Report Assembly : BusCreator  Inputs=4  OutDataTypeStr=Bus: MagnetometerReportBus  NonVirtualBus=on
  Report : Outport  InitialOutput=0
  wires:
  Measurement/1 -> Payload/1
  Payload/1 -> Report Assembly/1  "<B_B_T>"
  Payload/2 -> Report Assembly/2  "<valid>"
  Receipt Time/1 -> Report Assembly/3  "receive_time_s"
  Last Sequence/1 -> Next Sequence/1
  One/1 -> Next Sequence/2
  Next Sequence/1 -> Last Sequence/1, Report Assembly/4  "sequence_id"
  Report Assembly/1 -> Report/1

== system aocs_plant/Flight Dynamics/Orbit & Environment/Disturbance Torques ==
  AocsConfig : Inport
  EnvironmentConfig : Inport  Port=2
  AttitudeState : Inport  Port=3
  OrbitState : Inport  Port=4
  EnvironmentContext : Inport  Port=5
  SRP : Inport  Port=6
  MagneticField : Inport  Port=7
  Atmosphere : Inport  Port=8  OutDataTypeStr=Bus: AtmosphereBus
  Aerodynamic Disturbance Path : Subsystem
  Gravity Gradient Path : Subsystem
  Output Assembly : Subsystem
  Residual Magnetic Path : Subsystem
  SRP Disturbance Path : Subsystem
  Disturbance : Outport
  OrbitAcceleration : Outport  Port=2
  wires:
  AocsConfig/1 -> Aerodynamic Disturbance Path/4(AocsConfig), SRP Disturbance Path/3(AocsConfig), Gravity Gradient Path/3(AocsConfig)  "AocsConfig"
  EnvironmentConfig/1 -> Residual Magnetic Path/1(EnvironmentConfig), Gravity Gradient Path/5(EnvironmentConfig)
  MagneticField/1 -> Residual Magnetic Path/2(MagneticField)  "MagneticField"
  Atmosphere/1 -> Aerodynamic Disturbance Path/3(Atmosphere)  "Atmosphere"
  SRP/1 -> SRP Disturbance Path/1(SRP)  "SRP"
  Gravity Gradient Path/1(M_gg_B_Nm) -> Output Assembly/1(M_gg_B_Nm)  "M_gg_B_Nm"
  Residual Magnetic Path/1(M_rmm_B_Nm) -> Output Assembly/2(M_rmm_B_Nm)  "M_rmm_B_Nm"
  SRP Disturbance Path/1(M_srp_B_Nm) -> Output Assembly/3(M_srp_B_Nm)  "M_srp_B_Nm"
  Aerodynamic Disturbance Path/2(M_aero_B_Nm) -> Output Assembly/4(M_aero_B_Nm)  "M_aero_B_Nm"
  SRP Disturbance Path/2(F_srp_B_N) -> Output Assembly/5(F_srp_B_N)  "F_srp_B_N"
  SRP Disturbance Path/3(F_srp_I_N) -> Output Assembly/6(F_srp_I_N)  "F_srp_I_N"
  SRP Disturbance Path/4(a_srp_I_m_s2) -> Output Assembly/7(a_srp_I_m_s2)  "a_srp_I_m_s2"
  Aerodynamic Disturbance Path/1(F_aero_B_N) -> Output Assembly/8(F_aero_B_N)  "F_aero_B_N"
  Aerodynamic Disturbance Path/3(F_aero_I_N) -> Output Assembly/9(F_aero_I_N)  "F_aero_I_N"
  Aerodynamic Disturbance Path/4(a_aero_I_m_s2) -> Output Assembly/10(a_aero_I_m_s2)  "a_aero_I_m_s2"
  Aerodynamic Disturbance Path/5(q_dyn_N_m2) -> Output Assembly/11(q_dyn_N_m2)  "q_dyn_N_m2"
  Aerodynamic Disturbance Path/6(v_rel_norm_m_s) -> Output Assembly/12(v_rel_norm_m_s)  "v_rel_norm_m_s"
  Output Assembly/1(Disturbance) -> Disturbance/1  "Disturbance"
  Output Assembly/2(OrbitAcceleration) -> OrbitAcceleration/1  "a_dist_I_m_s2"
  EnvironmentContext/1 -> Gravity Gradient Path/4(EnvironmentContext)  "EnvironmentContext"
  OrbitState/1 -> Gravity Gradient Path/1(OrbitState), Aerodynamic Disturbance Path/1(OrbitState)  "OrbitState"
  AttitudeState/1 -> Aerodynamic Disturbance Path/2(AttitudeState), SRP Disturbance Path/2(AttitudeState), Gravity Gradient Path/2(AttitudeState)  "AttitudeState"

== system aocs_plant/Flight Dynamics/Orbit & Environment/Environment Bus Assembly ==
  Disturbance : Inport
  MagneticField : Inport  Port=2
  Sun : Inport  Port=3
  Illumination : Inport  Port=4
  Atmosphere : Inport  Port=5  OutDataTypeStr=Bus: AtmosphereBus
  Environment Bus Creator : BusCreator  Inputs=22  OutDataTypeStr=Bus: EnvironmentBus
  Select Disturbance : BusSelector  OutputSignals=M_dist_B_Nm,M_srp_B_Nm,F_srp_B_N,F_srp_I_N,a_srp_I_m_s2,M_aero_B_Nm,F_aero_B_N,F_aero_I_N,a_aero_I_m_s2,a_dist_I_m_s2,q_dyn_N_m2,v_rel_norm_m_s
  Select Illumination : BusSelector  OutputSignals=solar_flux_shadowed_W_m2,sun_visibility
  Select Magnetic Field : BusSelector  OutputSignals=B_I_T,B_B_T
  Select Sun : BusSelector  OutputSignals=sun_B_unit,sun_I_unit,r_sun_I_m,sun_distance_m,solar_flux_W_m2
  EnvironmentBus : Outport
  wires:
  Disturbance/1 -> Select Disturbance/1
  MagneticField/1 -> Select Magnetic Field/1
  Select Magnetic Field/1 -> Environment Bus Creator/2  "<B_I_T>"
  Select Magnetic Field/2 -> Environment Bus Creator/3  "<B_B_T>"
  Sun/1 -> Select Sun/1
  Select Sun/1 -> Environment Bus Creator/4  "<sun_B_unit>"
  Select Sun/2 -> Environment Bus Creator/5  "<sun_I_unit>"
  Select Sun/3 -> Environment Bus Creator/6  "<r_sun_I_m>"
  Select Sun/4 -> Environment Bus Creator/7  "<sun_distance_m>"
  Select Sun/5 -> Environment Bus Creator/8  "<solar_flux_W_m2>"
  Illumination/1 -> Select Illumination/1
  Select Illumination/1 -> Environment Bus Creator/9  "<solar_flux_shadowed_W_m2>"
  Select Illumination/2 -> Environment Bus Creator/10  "<sun_visibility>"
  Environment Bus Creator/1 -> EnvironmentBus/1  "EnvironmentBus"
  Atmosphere/1 -> Environment Bus Creator/11  "Atmosphere"
  Select Disturbance/1 -> Environment Bus Creator/1  "<M_dist_B_Nm>"
  Select Disturbance/2 -> Environment Bus Creator/12  "<M_srp_B_Nm>"
  Select Disturbance/3 -> Environment Bus Creator/13  "<F_srp_B_N>"
  Select Disturbance/4 -> Environment Bus Creator/14  "<F_srp_I_N>"
  Select Disturbance/5 -> Environment Bus Creator/15  "<a_srp_I_m_s2>"
  Select Disturbance/6 -> Environment Bus Creator/16  "<M_aero_B_Nm>"
  Select Disturbance/7 -> Environment Bus Creator/17  "<F_aero_B_N>"
  Select Disturbance/8 -> Environment Bus Creator/18  "<F_aero_I_N>"
  Select Disturbance/9 -> Environment Bus Creator/19  "<a_aero_I_m_s2>"
  Select Disturbance/10 -> Environment Bus Creator/20  "<a_dist_I_m_s2>"
  Select Disturbance/11 -> Environment Bus Creator/21  "<q_dyn_N_m2>"
  Select Disturbance/12 -> Environment Bus Creator/22  "<v_rel_norm_m_s>"

== system aocs_plant/Flight Dynamics/Orbit & Environment/Environment Products ==
  EnvironmentConfig : Inport
  AttitudeState : Inport  Port=2
  OrbitState : Inport  Port=3
  EnvironmentContext : Inport  Port=4
  Atmosphere Products : Subsystem
  Geomagnetic Field Model : Subsystem
  Illumination Model : Subsystem
  Solar Radiation Pressure : Subsystem
  Sun Products : Subsystem
  SRP : Outport
  MagneticField : Outport  Port=2
  Sun : Outport  Port=3
  Illumination : Outport  Port=4
  Atmosphere : Outport  Port=5  OutDataTypeStr=Bus: AtmosphereBus
  wires:
  Sun Products/1(Sun) -> Illumination Model/3(Sun), Solar Radiation Pressure/2(Sun), Sun/1
  Geomagnetic Field Model/1(MagneticField) -> MagneticField/1
  Solar Radiation Pressure/1(SRP) -> SRP/1  "SRP"
  OrbitState/1 -> Atmosphere Products/2(OrbitState), Sun Products/2(OrbitState), Illumination Model/1(OrbitState), Geomagnetic Field Model/3(OrbitState)
  Illumination Model/1(Illumination) -> Illumination/1, Solar Radiation Pressure/1(Illumination)
  EnvironmentConfig/1 -> Atmosphere Products/1(EnvironmentConfig), Illumination Model/2(EnvironmentConfig), Sun Products/1(EnvironmentConfig)
  EnvironmentContext/1 -> Sun Products/4(EnvironmentContext), Atmosphere Products/3(EnvironmentContext), Geomagnetic Field Model/2(EnvironmentContext)
  AttitudeState/1 -> Sun Products/3(AttitudeState), Geomagnetic Field Model/1(AttitudeState)
  Atmosphere Products/1(Atmosphere) -> Atmosphere/1

== system aocs_plant/Flight Dynamics/Orbit & Environment/Orbit Propagator & Time ==
  OrbitConfig : Inport
  OrbitAcceleration : Inport  Port=2
  Orbit State : Subsystem
  Orbit and Time Context : Subsystem
  OrbitState : Outport
  EnvironmentContext : Outport  Port=2
  wires:
  OrbitConfig/1 -> Orbit and Time Context/1(In1)
  Orbit State/1(OrbitState) -> OrbitState/1  "OrbitState"
  Orbit and Time Context/1(EnvironmentContext) -> EnvironmentContext/1  "EnvironmentContext"
  OrbitAcceleration/1 -> Orbit State/1(OrbitAcceleration)

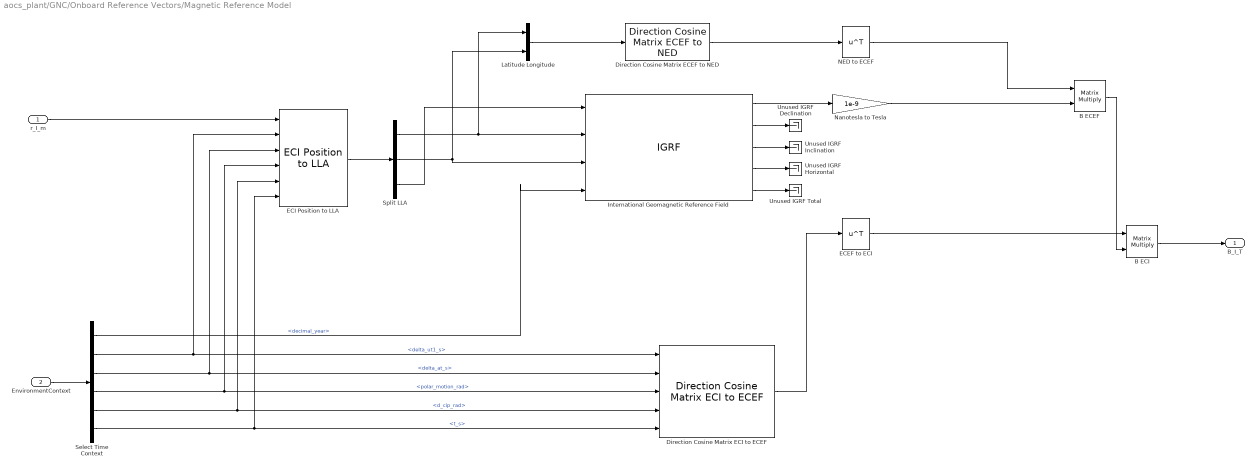
== system aocs_plant/GNC/Onboard Reference Vectors/Magnetic Reference Model ==
  r_I_m : Inport
  EnvironmentContext : Inport  Port=2  OutDataTypeStr=Bus: EnvironmentContextBus
  B ECEF : Product  Multiplication=Matrix(*)
  B ECI : Product  Multiplication=Matrix(*)
  Direction Cosine Matrix ECEF to NED : aerolibtransform2/Direction Cosine Matrix ECEF to NED
  Direction Cosine Matrix ECI to ECEF : aerolibtransform2/Direction Cosine Matrix ECI to ECEF  red=IAU-2000/2006  year=2026  month=January  day=1  hour=0  min=0  sec=0  deltaT=Sec  errorflag=Error  extraparamflag=on
      settings: AttributesFormatString=%<red>
  ECEF to ECI : Math  Operator=transpose
  ECI Position to LLA : aerolibtransform2/ECI Position to LLA  red=IAU-2000/2006  year=2026  month=January  day=1  hour=0  min=0  sec=0  deltaT=Sec  errorflag=Error  extraparamflag=on  eunits=Metric (MKS)  earthmodel=WGS84  flat=1/298.257223563  eqradius=6378137
      settings: AttributesFormatString=%<red>
  International Geomagnetic Reference Field : IGRF  month=January  day=1  sv_out=off
      settings: AttributesFormatString=%<generation>
  Latitude Longitude : Mux  Inputs=2
  NED to ECEF : Math  Operator=transpose
  Nanotesla to Tesla : Gain  Gain=1e-9
  Select Time Context : BusSelector  OutputSignals=decimal_year,delta_ut1_s,delta_at_s,polar_motion_rad,d_cip_rad,t_s
  Split LLA : Demux  Outputs=3
  Unused IGRF Declination : Terminator
  Unused IGRF Horizontal : Terminator
  Unused IGRF Inclination : Terminator
  Unused IGRF Total : Terminator
  B_I_T : Outport
  wires:
  EnvironmentContext/1 -> Select Time Context/1
  r_I_m/1 -> ECI Position to LLA/1
  Select Time Context/2 -> ECI Position to LLA/2, Direction Cosine Matrix ECI to ECEF/1  "<delta_ut1_s>"
  Select Time Context/3 -> ECI Position to LLA/3, Direction Cosine Matrix ECI to ECEF/2  "<delta_at_s>"
  Select Time Context/4 -> ECI Position to LLA/4, Direction Cosine Matrix ECI to ECEF/3  "<polar_motion_rad>"
  Select Time Context/5 -> ECI Position to LLA/5, Direction Cosine Matrix ECI to ECEF/4  "<d_cip_rad>"
  Select Time Context/6 -> ECI Position to LLA/6, Direction Cosine Matrix ECI to ECEF/5  "<t_s>"
  ECI Position to LLA/1 -> Split LLA/1
  Split LLA/3 -> International Geomagnetic Reference Field/1
  Split LLA/1 -> Latitude Longitude/1, International Geomagnetic Reference Field/2
  Split LLA/2 -> Latitude Longitude/2, International Geomagnetic Reference Field/3
  Select Time Context/1 -> International Geomagnetic Reference Field/4  "<decimal_year>"
  Latitude Longitude/1 -> Direction Cosine Matrix ECEF to NED/1
  Direction Cosine Matrix ECEF to NED/1 -> NED to ECEF/1
  International Geomagnetic Reference Field/1 -> Nanotesla to Tesla/1
  NED to ECEF/1 -> B ECEF/1
  Nanotesla to Tesla/1 -> B ECEF/2
  International Geomagnetic Reference Field/2 -> Unused IGRF Declination/1
  International Geomagnetic Reference Field/3 -> Unused IGRF Inclination/1
  International Geomagnetic Reference Field/4 -> Unused IGRF Horizontal/1
  International Geomagnetic Reference Field/5 -> Unused IGRF Total/1
  Direction Cosine Matrix ECI to ECEF/1 -> ECEF to ECI/1
  ECEF to ECI/1 -> B ECI/1
  B ECEF/1 -> B ECI/2
  B ECI/1 -> B_I_T/1

== system aocs_plant/GNC/Onboard Reference Vectors/Onboard Orbit Propagator (SGP4) ==
  CurrentTime : Inport
  Sgp4Config : Inport  Port=2  OutDataTypeStr=Bus: Sgp4ConfigBus
  Completed Updates : Rounding
  One Based Sequence : Bias  Bias=1  SaturateOnIntegerOverflow=off
  SGP4 : MATLABFcn  MATLABFcn=propagateOnboardSgp4(u)  OutputDimensions=7  Output1D=off  SampleTime=AOCS_GNCConfig.AttitudeInitialization.sgp4_sample_time_s
  SGP4 Clock : ZeroOrderHold  SampleTime=AOCS_GNCConfig.AttitudeInitialization.sgp4_sample_time_s
  SGP4 Inputs : Mux  Inputs=9
  Select SGP4 Config : BusSelector  OutputSignals=epoch_utc_jd,sgp4_semi_major_axis_m,sgp4_eccentricity,sgp4_inclination_deg,sgp4_raan_deg,sgp4_argument_of_periapsis_deg,sgp4_true_anomaly_deg,sgp4_bstar
  Sequence To Uint32 : DataTypeConversion  OutDataTypeStr=uint32  SaturateOnIntegerOverflow=off  RndMeth=Floor
  Split SGP4 State : Demux  Outputs=[3 3 1]
  Updates Elapsed : Gain  Gain=1/AOCS_GNCConfig.AttitudeInitialization.sgp4_sample_time_s
  r_I_m : Outport
  v_I_m_s : Outport  Port=2
  valid : Outport  Port=3
  update_time_s : Outport  Port=4
  sequence_id : Outport  Port=5
  wires:
  CurrentTime/1 -> SGP4 Clock/1
  SGP4 Clock/1 -> update_time_s/1, SGP4 Inputs/1, Updates Elapsed/1
  SGP4 Inputs/1 -> SGP4/1
  SGP4/1 -> Split SGP4 State/1
  Split SGP4 State/1 -> r_I_m/1
  Split SGP4 State/2 -> v_I_m_s/1
  Split SGP4 State/3 -> valid/1
  Updates Elapsed/1 -> Completed Updates/1
  Completed Updates/1 -> One Based Sequence/1
  One Based Sequence/1 -> Sequence To Uint32/1
  Sequence To Uint32/1 -> sequence_id/1
  Select SGP4 Config/1 -> SGP4 Inputs/2  "<epoch_utc_jd>"
  Select SGP4 Config/2 -> SGP4 Inputs/3  "<sgp4_semi_major_axis_m>"
  Select SGP4 Config/3 -> SGP4 Inputs/4  "<sgp4_eccentricity>"
  Select SGP4 Config/4 -> SGP4 Inputs/5  "<sgp4_inclination_deg>"
  Select SGP4 Config/5 -> SGP4 Inputs/6  "<sgp4_raan_deg>"
  Select SGP4 Config/6 -> SGP4 Inputs/7  "<sgp4_argument_of_periapsis_deg>"
  Select SGP4 Config/7 -> SGP4 Inputs/8  "<sgp4_true_anomaly_deg>"
  Select SGP4 Config/8 -> SGP4 Inputs/9  "<sgp4_bstar>"
  Sgp4Config/1 -> Select SGP4 Config/1
